simulink model "AdaptivelyControlledPendulum"  (R2023b)
settings: Solver=VariableStepAuto  StartTime=0.0  StopTime=2  FixedStep=0.01  RelTol=1e-3
model workspace (MAT data in the model file):
  I = Simulink.Parameter
  I.Value = 10
  I.DataType = 'auto'
  I.DocUnits = 'kg*m^2'
  I.Complexity = 'real'
  I.Dimensions = [1 1]
  MgL = Simulink.Parameter
  MgL.Value = 10
  MgL.DataType = 'auto'
  MgL.DocUnits = 'N*m'
  MgL.Complexity = 'real'
  MgL.Dimensions = [1 1]
  P = Simulink.Parameter
  P.Value = [1.8583  0.0125; 0.0125  0.0427]
  P.DataType = 'auto'
  P.Complexity = 'real'
  P.Dimensions = [2 2]
  k0 = Simulink.Parameter
  k0.Value = 40
  k0.DataType = 'auto'
  k0.Complexity = 'real'
  k0.Dimensions = [1 1]
  k1 = Simulink.Parameter
  k1.Value = 12
  k1.DataType = 'auto'
  k1.Complexity = 'real'
  k1.Dimensions = [1 1]
settings Model: Creator=frqbv  LastModifiedBy=anura

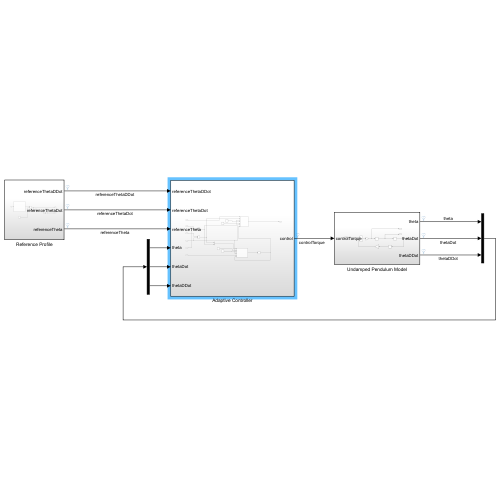
[thumbnail: Simulink's stored preview of the top-level diagram]
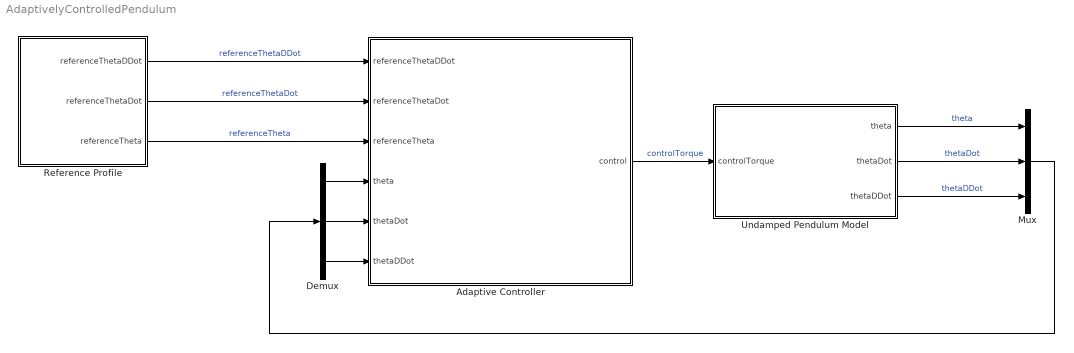
== system AdaptivelyControlledPendulum ==
  Adaptive Controller : Subsystem
  Demux : Demux  Outputs=3
  Mux : Mux  Inputs=3
  Reference Profile : Subsystem
  Undamped Pendulum Model : Subsystem
  wires:
  Undamped Pendulum Model/3(thetaDDot) -> Mux/3  "thetaDDot"
  Undamped Pendulum Model/1(theta) -> Mux/1  "theta"
  Undamped Pendulum Model/2(thetaDot) -> Mux/2  "thetaDot"
  Mux/1 -> Demux/1
  Reference Profile/1(referenceThetaDDot) -> Adaptive Controller/1(referenceThetaDDot)  "referenceThetaDDot"
  Reference Profile/2(referenceThetaDot) -> Adaptive Controller/2(referenceThetaDot)  "referenceThetaDot"
  Reference Profile/3(referenceTheta) -> Adaptive Controller/3(referenceTheta)  "referenceTheta"
  Demux/1 -> Adaptive Controller/4(theta)
  Demux/2 -> Adaptive Controller/5(thetaDot)
  Demux/3 -> Adaptive Controller/6(thetaDDot)
  Adaptive Controller/1(control) -> Undamped Pendulum Model/1(controlTorque)  "controlTorque"

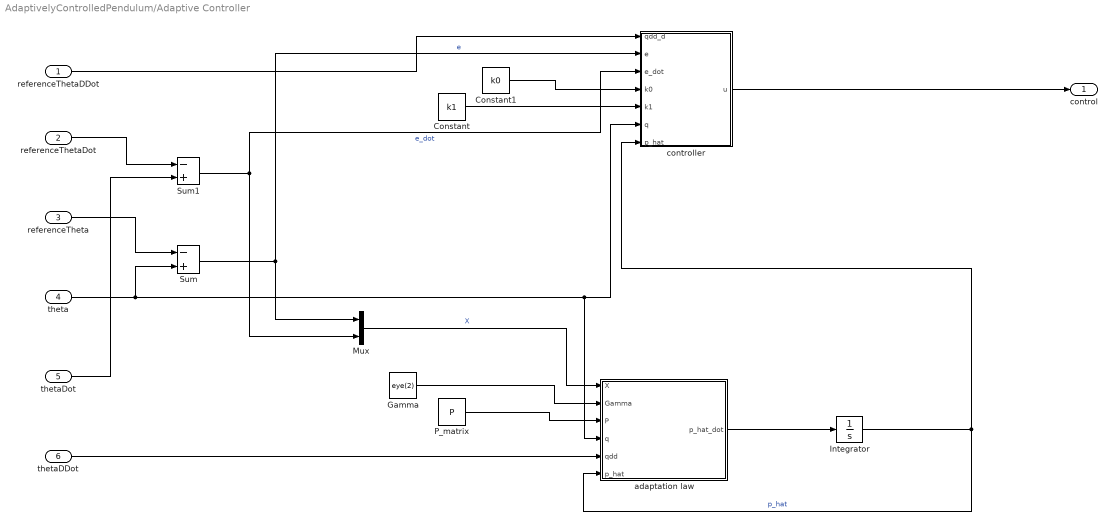
== system AdaptivelyControlledPendulum/Adaptive Controller ==
  referenceThetaDDot : Inport
  referenceThetaDot : Inport  Port=2
  referenceTheta : Inport  Port=3
  theta : Inport  Port=4
  thetaDot : Inport  Port=5
  thetaDDot : Inport  Port=6
  Constant : Constant  Value=k1
  Constant1 : Constant  Value=k0
  Gamma : Constant  Value=eye(2)
  Integrator : Integrator  InitialCondition=[8;5]
  Mux : Mux  Inputs=2
  P_matrix : Constant  Value=P
  Sum : Sum  Inputs=-+
  Sum1 : Sum  Inputs=-+
  adaptation law : MATLAB Function  TreatAsAtomicUnit=on
  controller : MATLAB Function  TreatAsAtomicUnit=on
  control : Outport
  wires:
  controller/1(u) -> control/1
  theta/1 -> controller/6(q), adaptation law/4(q), Sum/2
  referenceTheta/1 -> Sum/1
  referenceThetaDot/1 -> Sum1/1
  thetaDot/1 -> Sum1/2
  Sum1/1 -> controller/3(e_dot), Mux/2  "e_dot"
  Sum/1 -> controller/2(e), Mux/1  "e"
  P_matrix/1 -> adaptation law/3(P)
  Gamma/1 -> adaptation law/2(Gamma)
  adaptation law/1(p_hat_dot) -> Integrator/1
  Mux/1 -> adaptation law/1(X)  "X"
  Integrator/1 -> adaptation law/6(p_hat), controller/7(p_hat)  "p_hat"
  Constant/1 -> controller/5(k1)
  Constant1/1 -> controller/4(k0)
  referenceThetaDDot/1 -> controller/1(qdd_d)
  thetaDDot/1 -> adaptation law/5(qdd)

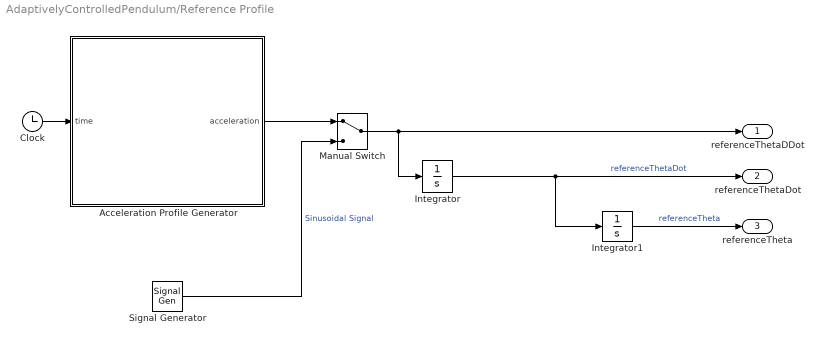
== system AdaptivelyControlledPendulum/Reference Profile ==
  Acceleration Profile Generator : MATLAB Function  TreatAsAtomicUnit=on
  Clock : Clock
  Integrator : Integrator
  Integrator1 : Integrator
  Manual Switch : ManualSwitch
  Signal Generator : SignalGenerator  Amplitude=2  Frequency=3
  referenceThetaDDot : Outport
  referenceThetaDot : Outport  Port=2
  referenceTheta : Outport  Port=3
  wires:
  Clock/1 -> Acceleration Profile Generator/1(time)
  Integrator/1 -> Integrator1/1, referenceThetaDot/1  "referenceThetaDot"
  Integrator1/1 -> referenceTheta/1  "referenceTheta"
  Signal Generator/1 -> Manual Switch/2  "Sinusoidal Signal"
  Acceleration Profile Generator/1(acceleration) -> Manual Switch/1
  Manual Switch/1 -> referenceThetaDDot/1, Integrator/1

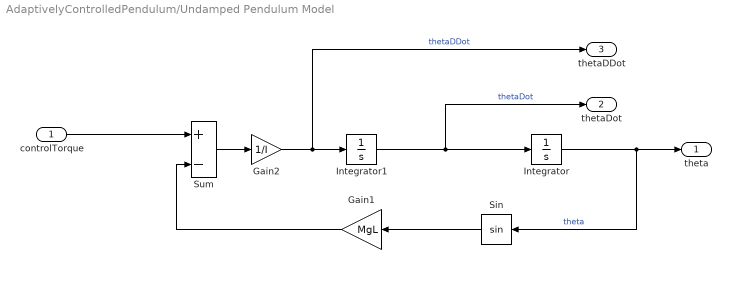
== system AdaptivelyControlledPendulum/Undamped Pendulum Model ==
  controlTorque : Inport
  Gain1 : Gain  Gain=MgL
  Gain2 : Gain  Gain=1/I
  Integrator : Integrator
  Integrator1 : Integrator
  Sin : Trigonometry
  Sum : Sum  Inputs=+-
  theta : Outport
  thetaDot : Outport  Port=2
  thetaDDot : Outport  Port=3
  wires:
  Integrator/1 -> Sin/1, theta/1  "theta"
  Integrator1/1 -> thetaDot/1, Integrator/1  "thetaDot"
  Sin/1 -> Gain1/1
  Gain1/1 -> Sum/2
  controlTorque/1 -> Sum/1
  Gain2/1 -> thetaDDot/1, Integrator1/1  "thetaDDot"
  Sum/1 -> Gain2/1

== matlab function AdaptivelyControlledPendulum/Adaptive Controller/adaptation law ==
  data: X input; p_hat_dot output; Gamma input; P input; q input; qdd input; p_hat input
function p_hat_dot = fcn(X, Gamma, P, q, qdd, p_hat)

B = [0;1];

y1 = qdd;
y2 = sin(q);

y = [y1,y2];

M_hat = p_hat(1);

Phi = (M_hat^(-1)) * y;

p_hat_dot = -Gamma^(-1) * (Phi') * (B') * (P) * (X);

== matlab function AdaptivelyControlledPendulum/Adaptive Controller/controller ==
  data: qdd_d input; u output; e input; e_dot input; k0 input; k1 input; q input; p_hat input
function u = fcn(qdd_d, e, e_dot, k0, k1, q, p_hat)

M_hat = p_hat(1);
mgl_hat = p_hat(2);

u = ((M_hat)*(qdd_d - (k0*e) - (k1*e_dot))) + (mgl_hat*sin(q));

== matlab function AdaptivelyControlledPendulum/Reference Profile/Acceleration Profile Generator ==
  data: time input; acceleration output
function acceleration = GenerateAccelerationProfile(time)

thetaMax = 1;
thetaDotMax = 1; 
thetaDoubleDotMax = 2;

t1 = thetaDotMax/thetaDoubleDotMax;
t2 = thetaMax / thetaDotMax;
t3 = t1 + t2;


if time <= t1
    acceleration = thetaDoubleDotMax;
elseif time <= t2
    acceleration = 0;
elseif time <= t3
    acceleration = -thetaDoubleDotMax;
else
    acceleration = 0;
end

end
